simulink model "Assignment1_V2"  (R2022b)
settings: Solver=FixedStepAuto  StartTime=0.0  StopTime=10.0  FixedStep=1e-3  RelTol=1e-3  EnableMultiTasking=on
undefined symbols (not defined in the file or in its folder): D0, D1, D10, D11, D12, D13, D2, D3, D4, D5, D6, D7, D8, D9, Pace_Mode, PTA0, PTA1, PTA2, PTB23, PTB9, PTC16, PTC17, PTC2, PTC3, PTC4, PTD0, PTD1, PTD2, PTD3
libraries: frdmk64flib x16, simulink x1
settings Model: ExtModeTrigDuration=5  Creator=a laptop  LastModifiedBy=a laptop
settings OptimizationCC: EnhancedBackFolding=on  PassReuseOutputArgsAs=Individual arguments  ZeroExternalMemoryAtStartup=off  ZeroInternalMemoryAtStartup=off  MaxStackSize=64  OptimizeBlockOrder=speed  DifferentSizesBufferReuse=on  OptimizationCustomize=off  EfficientTunableParamExpr=on
settings DebuggingCC: ParameterTunabilityLossMsg=error
settings HardwareCC: ProdBitPerPointer=32  ProdBitPerSizeT=32  ProdBitPerPtrDiffT=32  ProdLargestAtomicInteger=Long  ProdLargestAtomicFloat=Double  ProdWordSize=32  ProdHWDeviceType=ARM Compatible->ARM Cortex
settings ModelReferenceCC: EnableRefExpFcnMdlSchedulingChecks=on
settings SFSimCC: MATLABDynamicMemAlloc=off
settings RTWCC: Description=Embedded Coder  SystemTargetFile=ert.tlc  HardwareBoard=NXP FRDM-K64F  TLCOptions="-aInlineSetEventsForThisBaseRateFcn=TLC_FALSE -aSuppressMultiTaskScheduler=TLC_FALSE  -aRateBasedStepFcn=0"  TemplateMakefile=ert_default_tmf  Toolchain=GNU Tools for ARM Embedded Processors
settings CodeAppCC: ForceParamTrailComments=on  IgnoreCustomStorageClasses=off  OperatorAnnotations=on  SimulinkDataObjDesc=on  SFDataObjDesc=on  InsertBlockDesc=on
settings ERTTargetCC: ExtModeTransport=4  ExtModeMexFile=sendToCommService

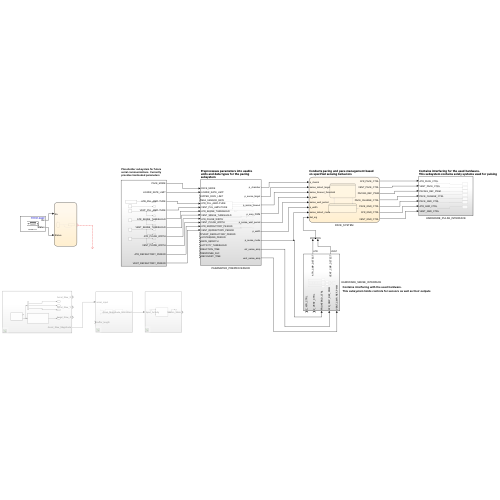
[thumbnail: Simulink's stored preview of the top-level diagram]
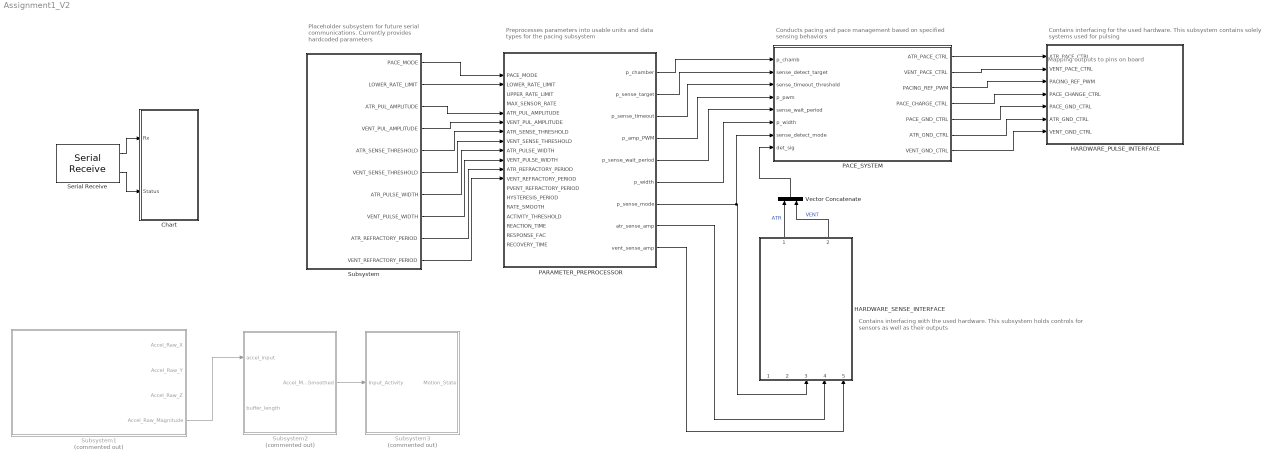
== system Assignment1_V2 ==
  note: Mapping outputs to pins on board
  note: Preprocesses parameters into usable units and data types for the pacing subsystem
  note: Conducts pacing and pace management based on specified sensing behaviors
  note: Contains interfacing for the used hardware.
      | This subsystem contains solely systems used for pulsing
  note: Placeholder subsystem for future serial communications. Currently provides hardcoded parameters
  note: Contains interfacing with the used hardware.
      | This subsystem holds controls for sensors as well as their outputs
  Chart : Stateflow chart  TreatAsAtomicUnit=on
  HARDWARE_PULSE_INTERFACE : Subsystem
  HARDWARE_SENSE_INTERFACE : Subsystem
  PACE_SYSTEM : Stateflow chart  TreatAsAtomicUnit=on
  PARAMETER_PREPROCESSOR : Subsystem
  Serial Receive : frdmk64flib/Serial Receive  SCIModule=0  Baudrate=uint32(9600)  Parity=None  StopBits=1  HardwareFlowControl=None  ByteOrder=LittleEndian  DataType=uint8  DataLength=10  BlockingMode=off  OutputStatus=on  SampleTime=-1
  Subsystem : Subsystem
  Subsystem1 : Subsystem  Commented=on
  Subsystem2 : Subsystem  Commented=on
  Subsystem3 : Subsystem  Commented=on
  Vector Concatenate : Concatenate
  wires:
  ? -> ?
  Serial Receive/1 -> Chart/1(Rx)
  PACE_SYSTEM/2(VENT_PACE_CTRL) -> HARDWARE_PULSE_INTERFACE/2(VENT_PACE_CTRL)
  Subsystem/7(ATR_PULSE_WIDTH) -> PARAMETER_PREPROCESSOR/9(ATR_PULSE_WIDTH)
  Subsystem1/4(Accel_Raw_Magnitude) -> Subsystem2/1(accel_input)
  Subsystem2/1(Accel_Magnitude_Smoothed) -> Subsystem3/1(Input_Activity)
  PARAMETER_PREPROCESSOR/3(p_sense_timeout) -> PACE_SYSTEM/3(sense_timeout_threshold)
  PACE_SYSTEM/5(PACE_GND_CTRL) -> HARDWARE_PULSE_INTERFACE/5(PACE_GND_CTRL)
  Subsystem/6(VENT_SENSE_THRESHOLD) -> PARAMETER_PREPROCESSOR/8(VENT_SENSE_THRESHOLD)
  PARAMETER_PREPROCESSOR/1(p_chamber) -> PACE_SYSTEM/1(p_chamb)
  Subsystem/9(ATR_REFRACTORY_PERIOD) -> PARAMETER_PREPROCESSOR/11(ATR_REFRACTORY_PERIOD)
  Subsystem/10(VENT_REFRACTORY_PERIOD) -> PARAMETER_PREPROCESSOR/12(VENT_REFRACTORY_PERIOD)
  HARDWARE_SENSE_INTERFACE/1(ATR_CMP_DETECT) -> Vector Concatenate/1  "ATR"
  PARAMETER_PREPROCESSOR/6(p_width) -> PACE_SYSTEM/6(p_width)
  PARAMETER_PREPROCESSOR/7(p_sense_mode) -> PACE_SYSTEM/7(sense_detect_mode), HARDWARE_SENSE_INTERFACE/3(FRONTEND_CTRL)
  Subsystem/8(VENT_PULSE_WIDTH) -> PARAMETER_PREPROCESSOR/10(VENT_PULSE_WIDTH)
  Serial Receive/2 -> Chart/2(Status)
  Subsystem/5(ATR_SENSE_THRESHOLD) -> PARAMETER_PREPROCESSOR/7(ATR_SENSE_THRESHOLD)
  Subsystem/3(ATR_PUL_AMPLITUDE) -> PARAMETER_PREPROCESSOR/5(ATR_PUL_AMPLITUDE)
  Subsystem/2(LOWER_RATE_LIMIT) -> PARAMETER_PREPROCESSOR/2(LOWER_RATE_LIMIT)
  PACE_SYSTEM/7(VENT_GND_CTRL) -> HARDWARE_PULSE_INTERFACE/7(VENT_GND_CTRL)
  HARDWARE_SENSE_INTERFACE/2(VENT_CMP_DETECT) -> Vector Concatenate/2  "VENT"
  PARAMETER_PREPROCESSOR/8(atr_sense_amp) -> HARDWARE_SENSE_INTERFACE/4(ATR_CMP_REF_PWM)
  PARAMETER_PREPROCESSOR/9(vent_sense_amp) -> HARDWARE_SENSE_INTERFACE/5(VENT_CMP_REF_PWM)
  Subsystem/1(PACE_MODE) -> PARAMETER_PREPROCESSOR/1(PACE_MODE)
  PARAMETER_PREPROCESSOR/4(p_amp_PWM) -> PACE_SYSTEM/4(p_pwm)
  PACE_SYSTEM/4(PACE_CHARGE_CTRL) -> HARDWARE_PULSE_INTERFACE/4(PACE_CHANGE_CTRL)
  PACE_SYSTEM/6(ATR_GND_CTRL) -> HARDWARE_PULSE_INTERFACE/6(ATR_GND_CTRL)
  PACE_SYSTEM/3(PACING_REF_PWM) -> HARDWARE_PULSE_INTERFACE/3(PACING_REF_PWM)
  Subsystem/4(VENT_PUL_AMPLITUDE) -> PARAMETER_PREPROCESSOR/6(VENT_PUL_AMPLITUDE)
  PARAMETER_PREPROCESSOR/5(p_sense_wait_period) -> PACE_SYSTEM/5(sense_wait_period)
  PARAMETER_PREPROCESSOR/2(p_sense_target) -> PACE_SYSTEM/2(sense_detect_target)
  Vector Concatenate/1 -> PACE_SYSTEM/8(det_sig)
  PACE_SYSTEM/1(ATR_PACE_CTRL) -> HARDWARE_PULSE_INTERFACE/1(ATR_PACE_CTRL)

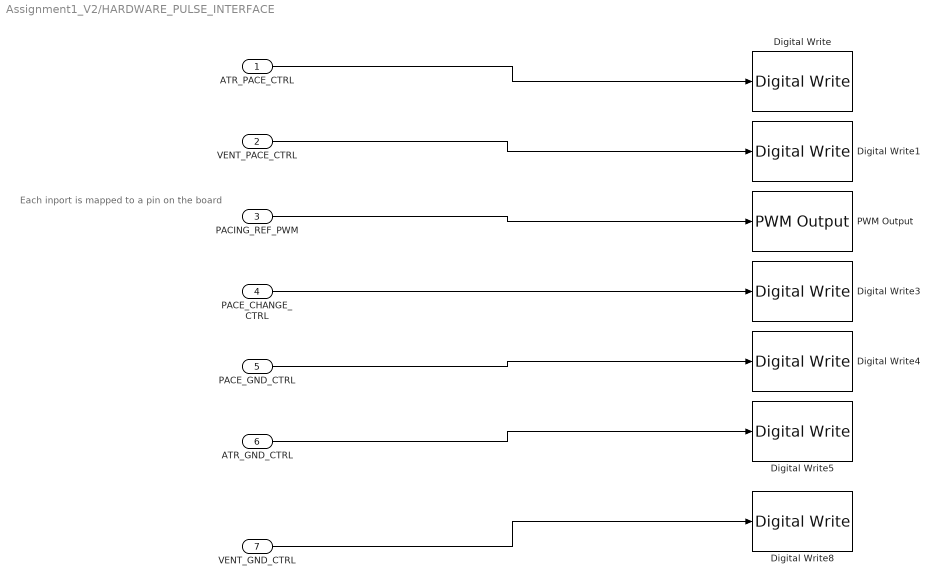
== system Assignment1_V2/HARDWARE_PULSE_INTERFACE ==
  note: Each inport is mapped to a pin on the board
  ATR_PACE_CTRL : Inport
  VENT_PACE_CTRL : Inport  Port=2
  PACING_REF_PWM : Inport  Port=3
  PACE_CHANGE_CTRL : Inport  Port=4
  PACE_GND_CTRL : Inport  Port=5
  ATR_GND_CTRL : Inport  Port=6
  VENT_GND_CTRL : Inport  Port=7
  Digital Write : frdmk64flib/Digital Write  Whichpin=PTA0 (D8)
  Digital Write1 : frdmk64flib/Digital Write  Whichpin=PTC4 (D9)
  Digital Write3 : frdmk64flib/Digital Write  Whichpin=PTB9 (D2)
  Digital Write4 : frdmk64flib/Digital Write  Whichpin=PTD0 (D10)
  Digital Write5 : frdmk64flib/Digital Write  Whichpin=PTD2 (D11)
  Digital Write8 : frdmk64flib/Digital Write  Whichpin=PTD3 (D12)
  PWM Output : frdmk64flib/PWM Output  Whichpin=PTA2 (D5)  InitialFrequency=2000  InitialDutyCycle=0
  wires:
  PACE_CHANGE_CTRL/1 -> Digital Write3/1
  PACE_GND_CTRL/1 -> Digital Write4/1
  VENT_PACE_CTRL/1 -> Digital Write1/1
  VENT_GND_CTRL/1 -> Digital Write8/1
  ATR_PACE_CTRL/1 -> Digital Write/1
  ATR_GND_CTRL/1 -> Digital Write5/1
  PACING_REF_PWM/1 -> PWM Output/1

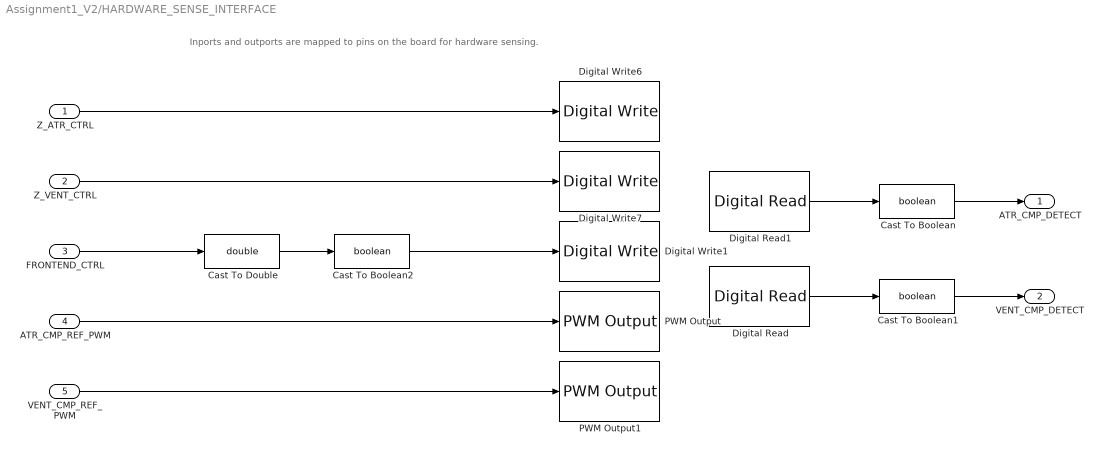
== system Assignment1_V2/HARDWARE_SENSE_INTERFACE ==
  note: Inports and outports are mapped to pins on the board for hardware sensing.
  Z_ATR_CTRL : Inport
  Z_VENT_CTRL : Inport  Port=2
  FRONTEND_CTRL : Inport  Port=3
  ATR_CMP_REF_PWM : Inport  Port=4
  VENT_CMP_REF_PWM : Inport  Port=5
  Cast To Boolean : DataTypeConversion  OutDataTypeStr=boolean  RndMeth=Round  SaturateOnIntegerOverflow=off
  Cast To Boolean1 : DataTypeConversion  OutDataTypeStr=boolean  RndMeth=Round  SaturateOnIntegerOverflow=off
  Cast To Boolean2 : DataTypeConversion  OutDataTypeStr=boolean  SaturateOnIntegerOverflow=off  RndMeth=Floor
  Cast To Double : DataTypeConversion  OutDataTypeStr=double  SaturateOnIntegerOverflow=off  RndMeth=Floor
  Digital Read : frdmk64flib/Digital Read  Whichpin=PTC17 (D1)  SampleTime=0.001
  Digital Read1 : frdmk64flib/Digital Read  Whichpin=PTC16 (D0)  SampleTime=0.001
  Digital Write1 : frdmk64flib/Digital Write  Whichpin=PTD1 (D13)
  Digital Write6 : frdmk64flib/Digital Write  Whichpin=PTB23 (D4)
  Digital Write7 : frdmk64flib/Digital Write  Whichpin=PTC3 (D7)
  PWM Output : frdmk64flib/PWM Output  Whichpin=PTC2 (D6)  InitialFrequency=2000  InitialDutyCycle=0
  PWM Output1 : frdmk64flib/PWM Output  Whichpin=PTA1 (D3)  InitialFrequency=2000  InitialDutyCycle=0
  ATR_CMP_DETECT : Outport  OutDataTypeStr=boolean
  VENT_CMP_DETECT : Outport  Port=2
  wires:
  Z_ATR_CTRL/1 -> Digital Write6/1
  Z_VENT_CTRL/1 -> Digital Write7/1
  FRONTEND_CTRL/1 -> Cast To Double/1
  ATR_CMP_REF_PWM/1 -> PWM Output/1
  VENT_CMP_REF_PWM/1 -> PWM Output1/1
  Digital Read1/1 -> Cast To Boolean/1
  Digital Read/1 -> Cast To Boolean1/1
  Cast To Boolean/1 -> ATR_CMP_DETECT/1
  Cast To Boolean1/1 -> VENT_CMP_DETECT/1
  Cast To Double/1 -> Cast To Boolean2/1
  Cast To Boolean2/1 -> Digital Write1/1

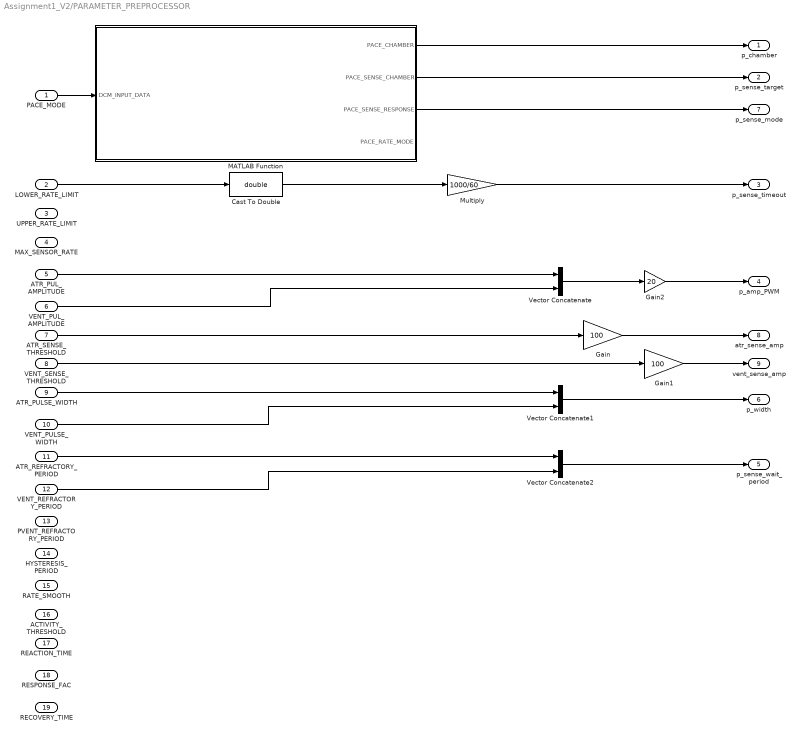
== system Assignment1_V2/PARAMETER_PREPROCESSOR ==
  PACE_MODE : Inport
  LOWER_RATE_LIMIT : Inport  Port=2
  UPPER_RATE_LIMIT : Inport  Port=3
  MAX_SENSOR_RATE : Inport  Port=4
  ATR_PUL_AMPLITUDE : Inport  Port=5
  VENT_PUL_AMPLITUDE : Inport  Port=6
  ATR_SENSE_THRESHOLD : Inport  Port=7
  VENT_SENSE_THRESHOLD : Inport  Port=8
  ATR_PULSE_WIDTH : Inport  Port=9
  VENT_PULSE_WIDTH : Inport  Port=10
  ATR_REFRACTORY_PERIOD : Inport  Port=11
  VENT_REFRACTORY_PERIOD : Inport  Port=12
  PVENT_REFRACTORY_PERIOD : Inport  Port=13
  HYSTERESIS_PERIOD : Inport  Port=14
  RATE_SMOOTH : Inport  Port=15
  ACTIVITY_THRESHOLD : Inport  Port=16
  REACTION_TIME : Inport  Port=17
  RESPONSE_FAC : Inport  Port=18
  RECOVERY_TIME : Inport  Port=19
  Cast To Double : DataTypeConversion  OutDataTypeStr=double  SaturateOnIntegerOverflow=off  RndMeth=Floor
  Gain : Gain  Gain=100
  Gain1 : Gain  Gain=100
  Gain2 : Gain  Gain=20
  MATLAB Function : MATLAB Function  TreatAsAtomicUnit=on
  Multiply : Gain  Gain=1000/60
  Vector Concatenate : Concatenate
  Vector Concatenate1 : Concatenate
  Vector Concatenate2 : Concatenate
  p_chamber : Outport
  p_sense_target : Outport  Port=2
  p_sense_timeout : Outport  Port=3
  p_amp_PWM : Outport  Port=4
  p_sense_wait_period : Outport  Port=5
  p_width : Outport  Port=6
  p_sense_mode : Outport  Port=7
  atr_sense_amp : Outport  Port=8
  vent_sense_amp : Outport  Port=9
  wires:
  PACE_MODE/1 -> MATLAB Function/1(DCM_INPUT_DATA)
  MATLAB Function/2(PACE_SENSE_CHAMBER) -> p_sense_target/1
  MATLAB Function/3(PACE_SENSE_RESPONSE) -> p_sense_mode/1
  LOWER_RATE_LIMIT/1 -> Cast To Double/1
  ATR_PUL_AMPLITUDE/1 -> Vector Concatenate/1
  VENT_PUL_AMPLITUDE/1 -> Vector Concatenate/2
  MATLAB Function/1(PACE_CHAMBER) -> p_chamber/1
  ATR_SENSE_THRESHOLD/1 -> Gain/1
  VENT_SENSE_THRESHOLD/1 -> Gain1/1
  Gain2/1 -> p_amp_PWM/1
  Vector Concatenate/1 -> Gain2/1
  ATR_PULSE_WIDTH/1 -> Vector Concatenate1/1
  VENT_PULSE_WIDTH/1 -> Vector Concatenate1/2
  Vector Concatenate1/1 -> p_width/1
  VENT_REFRACTORY_PERIOD/1 -> Vector Concatenate2/2
  Vector Concatenate2/1 -> p_sense_wait_period/1
  ATR_REFRACTORY_PERIOD/1 -> Vector Concatenate2/1
  Cast To Double/1 -> Multiply/1
  Multiply/1 -> p_sense_timeout/1
  Gain1/1 -> vent_sense_amp/1
  Gain/1 -> atr_sense_amp/1

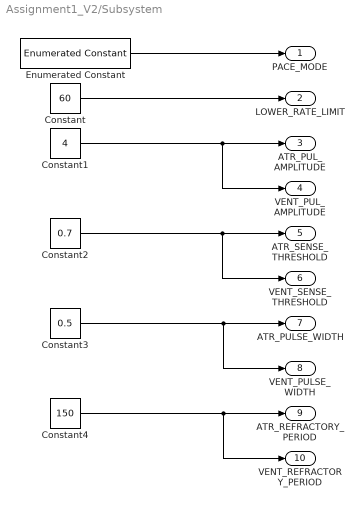
== system Assignment1_V2/Subsystem ==
  Constant : Constant  Value=60
  Constant1 : Constant  Value=4
  Constant2 : Constant  Value=0.7
  Constant3 : Constant  Value=0.5
  Constant4 : Constant  Value=150
  Enumerated Constant : simulink/Sources/Enumerated Constant  OutDataTypeStr=Enum: Pace_Mode  Value=Pace_Mode.AAI  SampleTime=inf
  PACE_MODE : Outport
  LOWER_RATE_LIMIT : Outport  Port=2
  ATR_PUL_AMPLITUDE : Outport  Port=3
  VENT_PUL_AMPLITUDE : Outport  Port=4
  ATR_SENSE_THRESHOLD : Outport  Port=5
  VENT_SENSE_THRESHOLD : Outport  Port=6
  ATR_PULSE_WIDTH : Outport  Port=7
  VENT_PULSE_WIDTH : Outport  Port=8
  ATR_REFRACTORY_PERIOD : Outport  Port=9
  VENT_REFRACTORY_PERIOD : Outport  Port=10
  wires:
  Enumerated Constant/1 -> PACE_MODE/1
  Constant/1 -> LOWER_RATE_LIMIT/1
  Constant1/1 -> VENT_PUL_AMPLITUDE/1, ATR_PUL_AMPLITUDE/1
  Constant2/1 -> VENT_SENSE_THRESHOLD/1, ATR_SENSE_THRESHOLD/1
  Constant3/1 -> VENT_PULSE_WIDTH/1, ATR_PULSE_WIDTH/1
  Constant4/1 -> VENT_REFRACTORY_PERIOD/1, ATR_REFRACTORY_PERIOD/1

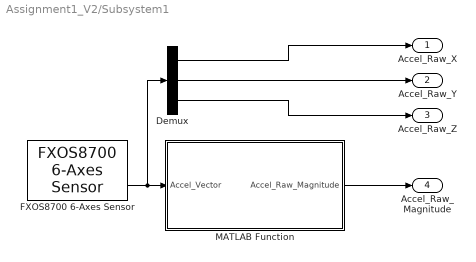
== system Assignment1_V2/Subsystem1 ==
  Demux : Demux  Outputs=3
  FXOS8700 6-Axes Sensor : frdmk64flib/FXOS8700 6-Axes Sensor  Activesensor=Accelerometer and Magnetometer  ODR=800Hz  HybridODR=400Hz  Accelfullrange=-4g to +4g  SampleTime=-1
  MATLAB Function : MATLAB Function  TreatAsAtomicUnit=on
  Accel_Raw_X : Outport
  Accel_Raw_Y : Outport  Port=2
  Accel_Raw_Z : Outport  Port=3
  Accel_Raw_Magnitude : Outport  Port=4
  wires:
  FXOS8700 6-Axes Sensor/2 -> MATLAB Function/1(Accel_Vector), Demux/1
  Demux/1 -> Accel_Raw_X/1
  Demux/2 -> Accel_Raw_Y/1
  Demux/3 -> Accel_Raw_Z/1
  MATLAB Function/1(Accel_Raw_Magnitude) -> Accel_Raw_Magnitude/1

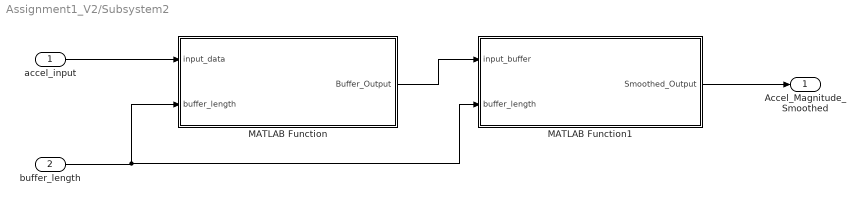
== system Assignment1_V2/Subsystem2 ==
  accel_input : Inport
  buffer_length : Inport  Port=2
  MATLAB Function : MATLAB Function  TreatAsAtomicUnit=on
  MATLAB Function1 : MATLAB Function  TreatAsAtomicUnit=on
  Accel_Magnitude_Smoothed : Outport
  wires:
  buffer_length/1 -> MATLAB Function1/2(buffer_length), MATLAB Function/2(buffer_length)
  accel_input/1 -> MATLAB Function/1(input_data)
  MATLAB Function/1(Buffer_Output) -> MATLAB Function1/1(input_buffer)
  MATLAB Function1/1(Smoothed_Output) -> Accel_Magnitude_Smoothed/1

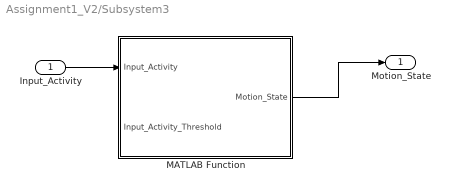
== system Assignment1_V2/Subsystem3 ==
  Input_Activity : Inport
  MATLAB Function : MATLAB Function  TreatAsAtomicUnit=on
  Motion_State : Outport
  wires:
  Input_Activity/1 -> MATLAB Function/1(Input_Activity)
  MATLAB Function/1(Motion_State) -> Motion_State/1

== matlab function Assignment1_V2/Subsystem2/MATLAB Function ==
  data: input_data input; Buffer_Output output; buffer_length input
function Buffer_Output = Generate_Buffer(input_data, buffer_length)
    Persistant Buffer_Internal;
    if (isempty(Buffer_Internal))
        Buffer_Internal = ones(buffer_length) * input_data;
    else
        for i = buffer_length-1:1
            Buffer_Internal[i+1] = Buffer_Internal[i]
        end
        Buffer_Internal[1] = input_data;
    end
    Buffer_Output = Buffer_Internal;
end

== matlab function Assignment1_V2/Subsystem2/MATLAB Function1 ==
  data: input_buffer input; Smoothed_Output output; buffer_length input
function Smoothed_Output = Smooth_Output(input_buffer, buffer_length)
    Sum_Value = 0;
    for i = Data_Array
        Sum_Value = Sum_Value + i;
    end
    Smoothed_Output = Sum_Value/buffer_length;
end

== matlab function Assignment1_V2/Subsystem3/MATLAB Function ==
  data: Input_Activity input; Motion_State output; Input_Activity_Threshold input
function Motion_State = Determine_Motion_State(Input_Activity, Input_Activity_Threshold)
    for i = 1:3
        if Input_Activity_Threshold[i] < Input_Activity
            Motion_State = Rate_Motion_State(i);
            return
        end
    end
end

== stateflow chart Assignment1_V2/Chart ==
  state Init
  state Decode
  (default) -> Init
  Init -> (junction 15)
  (junction 15) -> Decode : [Status == 0]
  Decode -> (junction 15)
  data: Rx input; Status input; Rx_D local

== matlab function Assignment1_V2/Subsystem1/MATLAB Function ==
  data: Accel_Vector input; Accel_Raw_Magnitude output
function Accel_Raw_Magnitude = Get_Magnitude(Accel_Vector)
    Accel_Raw_Magnitude = (Accel_Vector[1]^2 + Accel_Vector[2]^2 + Accel_Vector[3]^2)^(1/3);
end

== matlab function Assignment1_V2/PARAMETER_PREPROCESSOR/MATLAB Function ==
  data: DCM_INPUT_DATA input; PACE_CHAMBER output Enum: Pace_Chamber; PACE_SENSE_CHAMBER output Enum: Pace_Sense_Chamber; PACE_SENSE_RESPONSE output Enum: Pace_Sense_Response; PACE_RATE_MODE output Enum: Pace_Rate_Mode
function [PACE_CHAMBER, PACE_SENSE_CHAMBER, PACE_SENSE_RESPONSE, PACE_RATE_MODE] = Decode_Pacemode(DCM_INPUT_DATA)
    PACE_CHAMBER = Pace_Chamber(parse(DCM_INPUT_DATA,3));
    PACE_SENSE_CHAMBER = Pace_Sense_Chamber(parse(DCM_INPUT_DATA,2));
    PACE_SENSE_RESPONSE = Pace_Sense_Response(parse(DCM_INPUT_DATA,1));
    PACE_RATE_MODE = Pace_Rate_Mode(parse(DCM_INPUT_DATA,0));
end

function output = parse(DCM_INPUT_DATA, Bit_Depth)
    output = round((mod(double(DCM_INPUT_DATA), 10^(Bit_Depth+1)) - mod(double(DCM_INPUT_DATA), 10^Bit_Depth))/(10^Bit_Depth));
end

== stateflow chart Assignment1_V2/PACE_SYSTEM ==
  note: PACE sends pulses to the specified body part
  state PACE
    state Charge
      %Stop discharge of C22
      PACE_GND_CTRL = true;
      VENT_PACE_CTRL = false;
      ATR_PACE_CTRL = false;
      %Discharge blocking capacitor
      if p_chamb == Pace_Chamber.Atrium
      ATR_GND_CTRL = true;
      VENT_GND_CTRL = false;
      else
      ATR_GND_CTRL = false;
      VENT_GND_CTRL = true;
      end
      %Charge C22
      ATR_PACE_CTRL = false;
      VENT_PACE_CTRL = false;
      PACING_REF_PWM = p_pwm(double(p_chamb));
      PACE_CHARGE_CTRL = true;
      send(pace_compl)
    state Discharge_Prep
      %Prepares discharge
      %Stop charging C22
      PACING_REF_PWM = 0;
      PACE_CHARGE_CTRL = false;
      PACE_GND_CTRL = true;
      %Stop discharging blocking capacitor
      ATR_GND_CTRL = false;
      VENT_GND_CTRL = false;
    state Pace_Atr
      ATR_PACE_CTRL = true;
    state Pace_Vent
      VENT_PACE_CTRL = true;
    (default) -> Discharge_Prep
    Pace_Atr -> Charge : after(p_width(double(p_chamb)), msec)
    Discharge_Prep -> Pace_Atr [order 1] : [p_chamb == Pace_Chamber.Atrium]
    Discharge_Prep -> Pace_Vent [order 2] : [p_chamb == Pace_Chamber.Ventricle]
    Pace_Vent -> Charge : after(p_width(double(p_chamb)), msec)
  state SENSE
    state Sense_Finish
    state Sense_Disabled
      %All sensor timing is disabled
    state Sense_Wait
      %Sensor prep
    note: Warm-up period before sensor is active
    state Sense_Fail
      %Starts the pacing process
      send(sense_timeout)
    state Sense_Detect
      %Sensor active period
    state Sense_Detected
    note: This state is present for future DCM interactions and data logging
    (default) -> Sense_Finish
    Sense_Finish -> Sense_Disabled [order 2] : [sense_detect_mode == Pace_Sense_Response.Nothing]
    Sense_Finish -> Sense_Wait [order 1] : [sense_detect_mode ~= Pace_Sense_Response.Nothing]
    Sense_Disabled -> Sense_Fail : after(sense_timeout_threshold, msec)
    Sense_Detected -> Sense_Wait
    Sense_Wait -> Sense_Detect : after(sense_wait_period(double(sense_detect_target)), msec)
    Sense_Detect -> Sense_Fail [order 1] : [after(sense_timeout_threshold - sense_wait_period(double(sense_detect_target)), msec)]
    Sense_Detect -> Sense_Detected [order 2] : [det_sig(double(sense_detect_target)) == true]
  note: SENSE conducts all timing related operations and activates PACE when needed
  SENSE -> PACE : sense_timeout
  PACE -> SENSE : pace_compl
  (default) -> SENSE
  data: p_chamb input Enum: Pace_Chamber; sense_detect_target input; sense_timeout_threshold input double; p_pwm input; sense_wait_period input double; ATR_PACE_CTRL output; VENT_PACE_CTRL output; PACING_REF_PWM output; PACE_CHARGE_CTRL output; PACE_GND_CTRL output; ATR_GND_CTRL output; VENT_GND_CTRL output; p_width input double; sense_detect_mode input Enum: Pace_Sense_Response; det_sig input
  events: sense_timeout local FUNCTION_CALL_EVENT; pace_compl local FUNCTION_CALL_EVENT
